simulink model "PNMPTC_SSRP"  (R2018b)
settings: Solver=ode45  StartTime=0.0  StopTime=0.2  RelTol=1e-3
undefined symbols (not defined in the file): A, b, delta, lambda, omega, Tp, xi
settings Model: Creator=DELL  LastModifiedBy=DELL
settings DataIOCC: ExternalInput=[c1,c2,Pp,Tp]  InitialState=x0  LoadInitialState=on

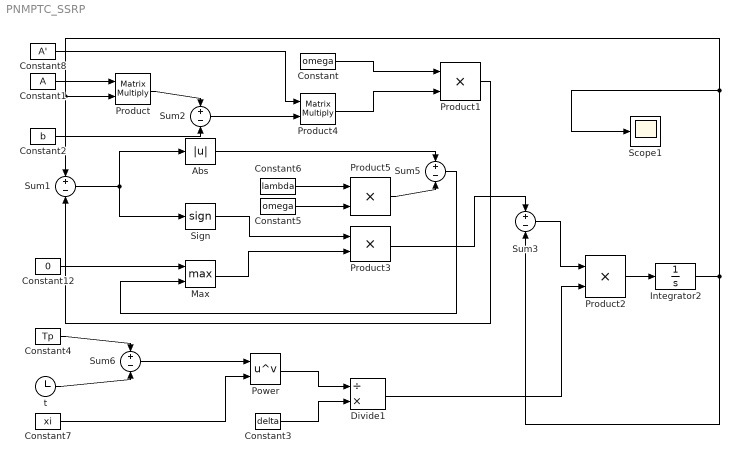
== system PNMPTC_SSRP ==
  Abs : Abs
  Constant : Constant  Value=omega
  Constant1 : Constant  Value=A
  Constant12 : Constant  Value=0
  Constant2 : Constant  Value=b
  Constant3 : Constant  Value=delta
  Constant4 : Constant  Value=Tp
  Constant5 : Constant  Value=omega
  Constant6 : Constant  Value=lambda
  Constant7 : Constant  Value=xi
  Constant8 : Constant  Value=A'
  Divide1 : Product  Inputs=/*
  Integrator2 : Integrator
  Max : MinMax  Function=max  Inputs=2
  Power : Math  Operator=pow  SaturateOnIntegerOverflow=on
  Product : Product  Multiplication=Matrix(*)
  Product{1..3,5} (4 alike) : Product
  Product4 : Product  Multiplication=Matrix(*)
  Scope1 : Scope
  Sign : Signum
  Sum{1..3,5..6} (5 alike) : Sum  Inputs=+-
  t : Clock
  wires:
  Constant12/1 -> Max/1
  Constant6/1 -> Product5/1
  Product5/1 -> Sum5/2
  Max/1 -> Product3/2
  Product/1 -> Sum2/1
  Abs/1 -> Sum5/1
  Constant5/1 -> Product5/2
  Constant2/1 -> Sum2/2
  Sum1/1 -> Abs/1, Sign/1
  Sign/1 -> Product3/1
  Constant1/1 -> Product/1
  Product1/1 -> Sum1/2
  Integrator2/1 -> Sum1/1, Product/2, Scope1/1, Sum3/2
  Sum5/1 -> Max/2
  Constant/1 -> Product1/1
  Product4/1 -> Product1/2
  Sum3/1 -> Product2/1
  Constant4/1 -> Sum6/1
  t/1 -> Sum6/2
  Sum6/1 -> Power/1
  Power/1 -> Divide1/1
  Constant3/1 -> Divide1/2
  Divide1/1 -> Product2/2
  Product2/1 -> Integrator2/1
  Product3/1 -> Sum3/1
  Constant8/1 -> Product4/1
  Sum2/1 -> Product4/2
  Constant7/1 -> Power/2
